simulink model "rocketExternalMeas"  (R2020b)
settings: Solver=FixedStepAuto  StartTime=0.0  StopTime=meas.t(end)  RelTol=1e-3
libraries: vrlib x3
settings Model: Creator=bean657  LastModifiedBy=Andreas

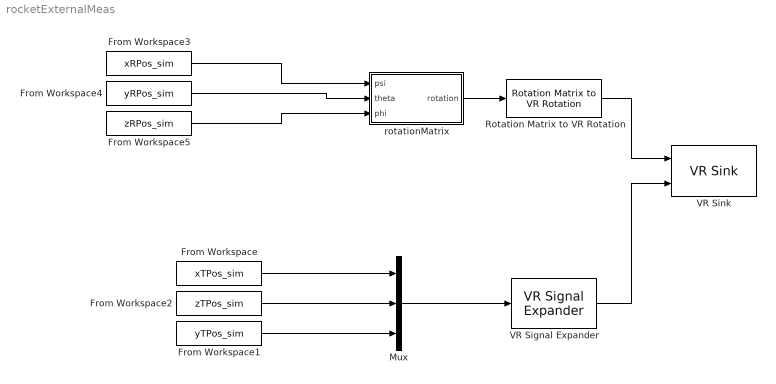
== system rocketExternalMeas ==
  From Workspace : FromWorkspace  VariableName=xTPos_sim
  From Workspace1 : FromWorkspace  VariableName=yTPos_sim
  From Workspace2 : FromWorkspace  VariableName=zTPos_sim
  From Workspace3 : FromWorkspace  VariableName=xRPos_sim
  From Workspace4 : FromWorkspace  VariableName=yRPos_sim
  From Workspace5 : FromWorkspace  VariableName=zRPos_sim
  Mux : Mux  Inputs=3
  Rotation Matrix to VR Rotation : vrlib/Utilities/Rotation Matrix to VR Rotation  maxzero=1e-12
      settings: SourceProductBaseCode=SL
  VR Signal Expander : vrlib/VR Signal Expander  outwidth=3  outidx=[1 2 3]
  VR Sink : vrlib/VR Sink  InstantiateOnLoad=on  SampleTime=0.1  ViewEnable=on  RemoteChange=off  RemoteView=off  FieldsWritten=Shuttle.rotation.4.1.1.double#Shuttle.translation.3.1.1.double  WorldFileName=rocketWorld.x3d  AutoView=off  VideoDimensions=[]  AllowVariableSize=off
  rotationMatrix : MATLAB Function  TreatAsAtomicUnit=on
  wires:
  VR Signal Expander/1 -> VR Sink/2
  rotationMatrix/1(rotation) -> Rotation Matrix to VR Rotation/1
  From Workspace3/1 -> rotationMatrix/1(psi)
  From Workspace4/1 -> rotationMatrix/2(theta)
  From Workspace5/1 -> rotationMatrix/3(phi)
  Rotation Matrix to VR Rotation/1 -> VR Sink/1
  Mux/1 -> VR Signal Expander/1
  From Workspace/1 -> Mux/1
  From Workspace2/1 -> Mux/2
  From Workspace1/1 -> Mux/3

== matlab function rocketExternalMeas/rotationMatrix ==
  data: psi input; rotation output; theta input; phi input
function rotation = fcn(psi,theta,phi)%yaw pitch roll

%yaw matrix
R3   = [ cos(psi) sin(psi) 0; 
             -sin(psi) cos(psi) 0; 
             0 0 1];
%pitch matrix
R2   = [cos(theta) 0 -sin(theta); 
        0  1           0; 
        sin(theta) 0  cos(theta)];
%roll matrix         
R1    = [1        0          0; 
         0  cos(phi)  sin(phi);
         0 -sin(phi)  cos(phi)];
         
         rotation = R1 * R2 * R3;
end
